simulink library "SimscapeCustomComponents_lib"  (R2025b)
settings: Solver=VariableStepAuto  StartTime=0.0  StopTime=10.0  RelTol=1e-3
undefined symbols (not defined in the file or in its folder): base, baseVdc, capacity, DiscIntNeverNeededParam, ee_sli_rtmsupport, filterInductance, freqeuncy, frequency, gcbh, gflInverter, gfmInverter, iMaxPU, Inertia, initialSOC, plantRating, solar, Ts, ups, Vac, windSystem, windTurbine
libraries: fl_lib x397, nesl_utility x171, eeGeneralControl x85, ee_lib x82, simulink x72, datacenter_lib x68, eeTransforms x38, slpidlib x24, buildingEnergy_lib x20, SimscapeFluids_lib x17, eeSinusoidalMeasurementV2 x8, eePwmGenerator x8
(part 13 of 24)

== system SimscapeCustomComponents_lib/Datacenter/PDU/PDU Racks (TL)/Server Tray (TL)/Server Tray ==
  AmbCPU : fl_lib/Thermal/Thermal Elements/Convective Heat Transfer  thermal_type=foundation.enum.constant_variable.constant  area=cpuSurfArea*nCPU m^2  heat_tr_coeff=htc W/(K*m^2)  min_heat_tr_coeff=1e-3 W/(K*m^2)  T_specify=off  T_priority=None  T=0 K  T_nominal_specify=off  T_nominal_value=1  T_nominal_unit=K  Q_specify=off  Q_priority=None  Q=0 W  Q_nominal_specify=off  Q_nominal_value=1  Q_nominal_unit=W
  AmbGPU : fl_lib/Thermal/Thermal Elements/Convective Heat Transfer  thermal_type=foundation.enum.constant_variable.constant  area=gpuSurfArea*nGPU m^2  heat_tr_coeff=htc W/(K*m^2)  min_heat_tr_coeff=1e-3 W/(K*m^2)  T_specify=off  T_priority=None  T=0 K  T_nominal_specify=off  T_nominal_value=1  T_nominal_unit=K  Q_specify=off  Q_priority=None  Q=0 W  Q_nominal_specify=off  Q_nominal_value=1  Q_nominal_unit=W
  PS Add : fl_lib/Physical Signals/Functions/PS Add
  Server Chip CPU : datacenter_lib/Server Chip  processorType=ProcessorType.CPU  numGPUs=4  numCPUs=nCPU  gpuTDP=1200 W  gpuIdlePower=300 W  gpuPowerExponent=1.4  hbmPowPerGPU=80 W  hbmUtilizationFrac=0.7  cpuTDP=cpuTDPperSocket W  cpuIdlePower=cpuIdlePower W  cpuPowerExponent=cpuExponent  PleakageCoeff=cpuLeakage W/K  chipTnominal=cpuNominalDieT K  chipCth=cpuDieThermalC J/K  T_specify=on  T_priority=High  T=initialT K  T_nominal_specify=off  T_nominal_value=1  T_nominal_unit=K  Q_specify=off  Q_priority=None  Q=0 W  Q_nominal_specify=off  Q_nominal_value=1  Q_nominal_unit=W
      settings: InternalSimscapePortConfiguration="{\"Bottom\":[{\"id\":\"H\",\"label\":\"H\",\"type\":\"foundation.thermal.thermal\"}],\"Left\":[{\"id\":\"U\",\"label\":\"U\",\"type\":\"input\"}],\"Right\":[{\"id\":\"Pow\",\"label\":\"P\",\"type\":\"output\"},{\"id\":\"Tchip\",\"label\":\"T\",\"type\":\"output\"}],\"Top\":[]}"
  Server Chip GPU : datacenter_lib/Server Chip  processorType=ProcessorType.GPU  numGPUs=nGPU  numCPUs=nCPU  gpuTDP=gpuTDPperDie W  gpuIdlePower=gpuIdlePower W  gpuPowerExponent=gpuExponent  hbmPowPerGPU=gpuHBMpower W  hbmUtilizationFrac=gpuHBMutil  cpuTDP=cpuTDPperSocket W  cpuIdlePower=cpuIdlePower W  cpuPowerExponent=1.1  PleakageCoeff=gpuLeakage W/K  chipTnominal=gpuNominalDieT K  chipCth=gpuDieThermalC J/K  T_specify=on  T_priority=High  T=initialT K  T_nominal_specify=off  T_nominal_value=1  T_nominal_unit=K  Q_specify=off  Q_priority=None  Q=0 W  Q_nominal_specify=off  Q_nominal_value=1  Q_nominal_unit=W
      settings: InternalSimscapePortConfiguration="{\"Bottom\":[{\"id\":\"H\",\"label\":\"H\",\"type\":\"foundation.thermal.thermal\"}],\"Left\":[{\"id\":\"U\",\"label\":\"U\",\"type\":\"input\"}],\"Right\":[{\"id\":\"Pow\",\"label\":\"P\",\"type\":\"output\"},{\"id\":\"Tchip\",\"label\":\"T\",\"type\":\"output\"}],\"Top\":[]}"
  TR_CPU_Amb : fl_lib/Thermal/Thermal Elements/Thermal Resistance  resistance=cpuAmbientR/nCPU K/W  T_specify=off  T_priority=None  T=0 K  T_nominal_specify=off  T_nominal_value=1  T_nominal_unit=K  Q_specify=off  Q_priority=None  Q=0 W  Q_nominal_specify=off  Q_nominal_value=1  Q_nominal_unit=W
  TR_CPU_substrate : fl_lib/Thermal/Thermal Elements/Thermal Resistance  resistance=cpuHeatSinkR/nCPU K/W  T_specify=off  T_priority=None  T=0 K  T_nominal_specify=off  T_nominal_value=1  T_nominal_unit=K  Q_specify=off  Q_priority=None  Q=0 W  Q_nominal_specify=off  Q_nominal_value=1  Q_nominal_unit=W
  TR_GPU_Amb : fl_lib/Thermal/Thermal Elements/Thermal Resistance  resistance=gpuAmbientR/nGPU K/W  T_specify=off  T_priority=None  T=0 K  T_nominal_specify=off  T_nominal_value=1  T_nominal_unit=K  Q_specify=off  Q_priority=None  Q=0 W  Q_nominal_specify=off  Q_nominal_value=1  Q_nominal_unit=W
  TR_GPU_substrate : fl_lib/Thermal/Thermal Elements/Thermal Resistance  resistance=gpuHeatSinkR/nGPU K/W  T_specify=off  T_priority=None  T=0 K  T_nominal_specify=off  T_nominal_value=1  T_nominal_unit=K  Q_specify=off  Q_priority=None  Q=0 W  Q_nominal_specify=off  Q_nominal_value=1  Q_nominal_unit=W
  TR_Tray_Amb : fl_lib/Thermal/Thermal Elements/Thermal Resistance  resistance=trayThermalR K/W  T_specify=off  T_priority=None  T=0 K  T_nominal_specify=off  T_nominal_value=1  T_nominal_unit=K  Q_specify=off  Q_priority=None  Q=0 W  Q_nominal_specify=off  Q_nominal_value=1  Q_nominal_unit=W
  Tray Thermal Mass : fl_lib/Thermal/Thermal Elements/Thermal Mass  mass_type=foundation.enum.constant_variable.constant  mass=trayMass kg  sp_heat=trayCp J/(K*kg)  mass_min=1e-6 kg  num_ports=foundation.enum.numPorts2.two  m_specify=off  m_priority=High  m=1 kg  m_nominal_specify=off  m_nominal_value=1  m_nominal_unit=kg  T_specify=on  T_priority=High  T=initialT K  T_nominal_specify=off  T_nominal_value=1  T_nominal_unit=K  Q_specify=off  Q_priority=None  Q=0 W  Q_nominal_specify=off  Q_nominal_value=1  Q_nominal_unit=W
      settings: InternalSimscapePortConfiguration="{\"Bottom\":[],\"Left\":[{\"id\":\"M\",\"label\":\"\",\"type\":\"foundation.thermal.thermal\"}],\"Right\":[{\"id\":\"N\",\"label\":\"\",\"type\":\"foundation.thermal.thermal\"}],\"Top\":[]}"
  U_gpu : PMIOPort  Side=Left
  U_cpu : PMIOPort  Port=2  Side=Left
  P : PMIOPort  Port=3  Side=Right
  T_gpu : PMIOPort  Port=4  Side=Right
  T_cpu : PMIOPort  Port=5  Side=Right
  Hc : PMIOPort  Port=6  Side=Right
  Ha : PMIOPort  Port=7  Side=Left
  connections:
  AmbCPU/LConn1 -- TR_CPU_Amb/RConn1
  PS Add/LConn2 -- Server Chip CPU/RConn1
  PS Add/LConn1 -- Server Chip GPU/RConn1
  P/RConn1 -- PS Add/RConn1
  Ha/RConn1 -- AmbGPU/RConn1 -- AmbCPU/RConn1
  AmbGPU/LConn1 -- TR_GPU_Amb/LConn1
  TR_Tray_Amb/RConn1 -- Hc/RConn1
  Server Chip CPU/RConn2 -- T_cpu/RConn1
  Server Chip CPU/LConn1 -- U_cpu/RConn1
  Server Chip GPU/LConn1 -- U_gpu/RConn1
  TR_Tray_Amb/LConn1 -- Tray Thermal Mass/RConn1
  TR_GPU_substrate/LConn1 -- Server Chip GPU/RConn3 -- TR_GPU_Amb/RConn1
  Server Chip CPU/RConn3 -- TR_CPU_Amb/LConn1 -- TR_CPU_substrate/LConn1
  Server Chip GPU/RConn2 -- T_gpu/RConn1
  TR_CPU_substrate/RConn1 -- TR_GPU_substrate/RConn1 -- Tray Thermal Mass/LConn1

== system SimscapeCustomComponents_lib/Microgrid and Renewables/Control/BESS/Grid Following Control/Current_controller ==
  id-ref : Inport
  ipvd : Inport  Port=2
  iqref : Inport  Port=3
  iq : Inport  Port=4
  Vd : Inport  Port=5
  Vq : Inport  Port=6
  Constant4 : Constant  Value=0
  Gain1 : Gain  Gain=2*1*pi*frequency*L/zbase
  Gain2 : Gain  Gain=2*1*pi*frequency*L/zbase
  Mux1 : Mux  Inputs=3
  PID Controller : slpidlib/PID Controller  Controller=PID  Form=Parallel  TimeDomain=Discrete-time  UseExternalTs=off  SampleTime=-1  IntegratorMethod=Forward Euler  FilterMethod=Forward Euler  ControllerParametersSource=internal  P=Kpic  I=Kiic  UseKiTs=off  D=Kd  UseExternalDerivativeSource=off  N=100  UseFilter=on  TunerSelectOption=Transfer Function Based (PID Tuner App)  InitialConditionSource=internal  InitialConditionForIntegrator=0  InitialConditionForFilter=0  DifferentiatorICPrevScaledInput=0  ExternalReset=none  TrackingMode=off  Kt=1  LimitOutput=off  SatLimitsSource=internal  UpperSaturationLimit=inf  LowerSaturationLimit=-inf  LinearizeAsGain=on  AntiWindupMode=none  Kb=1  LimitIntegrator=off  UpperIntegratorSaturationLimit=inf  LowerIntegratorSaturationLimit=-inf  POutMin=[]  POutMax=[]  IOutMin=[]  IOutMax=[]  DOutMin=[]  DOutMax=[]  NOutMin=[]  NOutMax=[]  SumOutMin=[]  SumOutMax=[]  SaturationOutMin=[]  SaturationOutMax=[]  PParamMin=[]  PParamMax=[]  IParamMin=[]  IParamMax=[]  DParamMin=[]  DParamMax=[]  NParamMin=[]  NParamMax=[]  KbParamMin=[]  KbParamMax=[]  KtParamMin=[]  KtParamMax=[]  KbOutMin=[]  KbOutMax=[]  KtOutMin=[]  KtOutMax=[]  IntegratorOutMin=[]  IntegratorOutMax=[]  FilterOutMin=[]  FilterOutMax=[]  SumI1OutMin=[]  SumI1OutMax=[]  SumI2OutMin=[]  SumI2OutMax=[]  SumI3OutMin=[]  SumI3OutMax=[]  SumI4OutMin=[]  SumI4OutMax=[]  SumDOutMin=[]  SumDOutMax=[]  DifferentiatorOutMin=[]  DifferentiatorOutMax=[]  FilterDiffOutCoefMin=[]  FilterDiffOutCoefMax=[]  ReciprocalOutMin=[]  ReciprocalOutMax=[]  SumDenOutMin=[]  SumDenOutMax=[]  SumNumOutMin=[]  SumNumOutMax=[]  DivideOutMin=[]  DivideOutMax=[]  UdiffTsProdOutMin=[]  UdiffTsProdOutMax=[]  NTsProdOutMin=[]  NTsProdOutMax=[]  UintegralTsProdOutMin=[]  UintegralTsProdOutMax=[]  UngainTsProdOutMin=[]  UngainTsProdOutMax=[]  ClampingZeroOutDataTypeStr=Inherit: Inherit via back propagation  ClampingZeroOutMin=[]  ClampingZeroOutMax=[]  FilterDenConstantOutDataTypeStr=Inherit: Inherit via back propagation  FilterDenConstantOutMin=[]  FilterDenConstantOutMax=[]  PCopyOutDataTypeStr=Inherit: Inherit via back propagation  PCopyOutMin=[]  PCopyOutMax=[]  NCopyOutDataTypeStr=Inherit: Inherit via back propagation  NCopyOutMin=[]  NCopyOutMax=[]  IntegratorContinuousStateAttributes=''  IntegratorStateMustResolveToSignalObject=off  IntegratorRTWStateStorageClass=Auto  FilterContinuousStateAttributes=''  FilterStateMustResolveToSignalObject=off  FilterRTWStateStorageClass=Auto  ParallelPVariant=InternalParameters  IdealPVariant=Disabled  IVariant=InternalParameters  DVariant=InternalParameters  IntegratorVariant=Discrete  SatVariant=Disabled  AWVariant=Passthrough  PCopyVariant=Disabled  TRVariant=Disabled  FdbkBlocksVariant=Forward  IdealPFdbkVariant=Disabled  SatFdbkVariant=Disabled  DerivativeFilterVariant=ForwardEulerFilter  NVariant=InternalParameters  NCopyVariant=Disabled  FilterICVariant=InternalICsFilter  IntegratorICVariant=InternalICs  ExternalResetVariant=Disabled  TRSumVariant=Passthrough  SumFdbkVariant=Disabled  SumVariant=Sum_PID  TsampFilterVariant=InternalTs  TsampNgainVariant=Passthrough  TsampIntegralVariant=Disabled_SignalSpec  ExternalSaturationOutDataTypeStr=Inherit: Same as second input  DerivativeSourceVariant=ErrorSignal  PreIntVariant=InternalPreInt
  PID Controller1 : slpidlib/PID Controller  Controller=PID  Form=Parallel  TimeDomain=Discrete-time  UseExternalTs=off  SampleTime=-1  IntegratorMethod=Forward Euler  FilterMethod=Forward Euler  ControllerParametersSource=internal  P=Kpic  I=Kiic  UseKiTs=off  D=Kd  UseExternalDerivativeSource=off  N=100  UseFilter=on  TunerSelectOption=Transfer Function Based (PID Tuner App)  InitialConditionSource=internal  InitialConditionForIntegrator=0  InitialConditionForFilter=0  DifferentiatorICPrevScaledInput=0  ExternalReset=none  TrackingMode=off  Kt=1  LimitOutput=off  SatLimitsSource=internal  UpperSaturationLimit=inf  LowerSaturationLimit=-inf  LinearizeAsGain=on  AntiWindupMode=none  Kb=1  LimitIntegrator=off  UpperIntegratorSaturationLimit=inf  LowerIntegratorSaturationLimit=-inf  POutMin=[]  POutMax=[]  IOutMin=[]  IOutMax=[]  DOutMin=[]  DOutMax=[]  NOutMin=[]  NOutMax=[]  SumOutMin=[]  SumOutMax=[]  SaturationOutMin=[]  SaturationOutMax=[]  PParamMin=[]  PParamMax=[]  IParamMin=[]  IParamMax=[]  DParamMin=[]  DParamMax=[]  NParamMin=[]  NParamMax=[]  KbParamMin=[]  KbParamMax=[]  KtParamMin=[]  KtParamMax=[]  KbOutMin=[]  KbOutMax=[]  KtOutMin=[]  KtOutMax=[]  IntegratorOutMin=[]  IntegratorOutMax=[]  FilterOutMin=[]  FilterOutMax=[]  SumI1OutMin=[]  SumI1OutMax=[]  SumI2OutMin=[]  SumI2OutMax=[]  SumI3OutMin=[]  SumI3OutMax=[]  SumI4OutMin=[]  SumI4OutMax=[]  SumDOutMin=[]  SumDOutMax=[]  DifferentiatorOutMin=[]  DifferentiatorOutMax=[]  FilterDiffOutCoefMin=[]  FilterDiffOutCoefMax=[]  ReciprocalOutMin=[]  ReciprocalOutMax=[]  SumDenOutMin=[]  SumDenOutMax=[]  SumNumOutMin=[]  SumNumOutMax=[]  DivideOutMin=[]  DivideOutMax=[]  UdiffTsProdOutMin=[]  UdiffTsProdOutMax=[]  NTsProdOutMin=[]  NTsProdOutMax=[]  UintegralTsProdOutMin=[]  UintegralTsProdOutMax=[]  UngainTsProdOutMin=[]  UngainTsProdOutMax=[]  ClampingZeroOutDataTypeStr=Inherit: Inherit via back propagation  ClampingZeroOutMin=[]  ClampingZeroOutMax=[]  FilterDenConstantOutDataTypeStr=Inherit: Inherit via back propagation  FilterDenConstantOutMin=[]  FilterDenConstantOutMax=[]  PCopyOutDataTypeStr=Inherit: Inherit via back propagation  PCopyOutMin=[]  PCopyOutMax=[]  NCopyOutDataTypeStr=Inherit: Inherit via back propagation  NCopyOutMin=[]  NCopyOutMax=[]  IntegratorContinuousStateAttributes=''  IntegratorStateMustResolveToSignalObject=off  IntegratorRTWStateStorageClass=Auto  FilterContinuousStateAttributes=''  FilterStateMustResolveToSignalObject=off  FilterRTWStateStorageClass=Auto  ParallelPVariant=InternalParameters  IdealPVariant=Disabled  IVariant=InternalParameters  DVariant=InternalParameters  IntegratorVariant=Discrete  SatVariant=Disabled  AWVariant=Passthrough  PCopyVariant=Disabled  TRVariant=Disabled  FdbkBlocksVariant=Forward  IdealPFdbkVariant=Disabled  SatFdbkVariant=Disabled  DerivativeFilterVariant=ForwardEulerFilter  NVariant=InternalParameters  NCopyVariant=Disabled  FilterICVariant=InternalICsFilter  IntegratorICVariant=InternalICs  ExternalResetVariant=Disabled  TRSumVariant=Passthrough  SumFdbkVariant=Disabled  SumVariant=Sum_PID  TsampFilterVariant=InternalTs  TsampNgainVariant=Passthrough  TsampIntegralVariant=Disabled_SignalSpec  ExternalSaturationOutDataTypeStr=Inherit: Same as second input  DerivativeSourceVariant=ErrorSignal  PreIntVariant=InternalPreInt
  Scope : Scope  NumInputPorts=2
      settings: ActiveDisplayYMinimum=-1  ActiveDisplayYMaximum=1
  Scope1 : Scope  NumInputPorts=2
      settings: ActiveDisplayYMinimum=-1.21282  ActiveDisplayYMaximum=0.9154  DataLoggingVariableName=ScopeData2
  Sum1 : Sum  Inputs=|+-
  Sum3 : Sum  Inputs=|++-
  Sum4 : Sum  Inputs=|+++
  Sum5 : Sum  Inputs=|+-
  mdq0 : Outport
  wires:
  PID Controller/1 -> Sum3/2
  Sum3/1 -> Mux1/1, [Ed]
  Gain2/1 -> Sum3/3
  ipvd/1 -> Scope/2, Gain1/1, Sum1/2
  id-ref/1 -> Scope/1, Sum1/1
  Gain1/1 -> Sum4/3
  Vq/1 -> Sum4/2
  iq/1 -> Scope1/2, Gain2/1, Sum5/2
  Sum1/1 -> PID Controller/1
  Vd/1 -> Sum3/1
  Constant4/1 -> Mux1/3
  Sum5/1 -> PID Controller1/1
  PID Controller1/1 -> Sum4/1
  Sum4/1 -> Mux1/2, [Eq]
  Mux1/1 -> mdq0/1
  iqref/1 -> Scope1/1, Sum5/1

== system SimscapeCustomComponents_lib/Microgrid and Renewables/Control/BESS/Grid Following Control/Reference Current ==
  note: Current Limiters
  note: Avoid division by zero during start
  V_ref : Inport
  V-mag : Inport  Port=2
  del f : Inport  Port=3
  LVRT_iq : Inport  Port=4
  PRef : Inport  Port=5
  QRef : Inport  Port=6
  Constant1 : Constant
  Constant3 : Constant  Value=Imax
  Current limits : Subsystem
  Refernce id generation : Subsystem
  Refernce iq generation : Subsystem
  Switch : Switch  Criteria=u2 ~= 0  SaturateOnIntegerOverflow=off  InputSameDT=off
  Unit Delay1 : UnitDelay  SampleTime=Ts
  Unit Delay3 : UnitDelay  SampleTime=Ts
  id_ref : Outport
  iq_ref : Outport  Port=2
  wires:
  Unit Delay1/1 -> Current limits/2(iqref)
  Current limits/1(iubq) -> Refernce iq generation/1(ubiq)
  Unit Delay3/1 -> Current limits/3(idref)
  Constant3/1 -> Current limits/1(Imax)
  Refernce id generation/1(id_ref) -> id_ref/1, Unit Delay3/1
  del f/1 -> Refernce id generation/2(del f)
  V_ref/1 -> Refernce iq generation/2(V_ref)
  Refernce iq generation/1(iq_ref) -> Unit Delay1/1, iq_ref/1
  LVRT_iq/1 -> Refernce iq generation/4(LVRT_iq)
  V-mag/1 -> Switch/1, Switch/2
  Switch/1 -> Refernce id generation/1(V_mag), Refernce iq generation/3(V_mag)
  Constant1/1 -> Switch/3
  QRef/1 -> Refernce iq generation/5(Q_ref)
  PRef/1 -> Refernce id generation/4(PRef)
  Current limits/2(iubd) -> Refernce id generation/3(ubid)

== system SimscapeCustomComponents_lib/Microgrid and Renewables/Control/BESS/Grid Forming Control/Current Limiting ==
  In Bus Element : Inport  PortName=measure  Element=Igd
  In Bus Element1 : Inport  PortName=measure  Element=Igq
  In Bus Element2 : Inport  Port=2  PortName=reactiveControl  Element=Vmd
  In Bus Element4 : Inport  Port=2  PortName=reactiveControl  Element=Vmq
  CurrentLimitingMethod : Subsystem  Variant=on  VariantControlMode=label  VariantControl=Choice  LabelModeActiveChoice=ctSat
  Scope : Scope  NumInputPorts=2
  Subtract : Sum  Inputs=+-
  Subtract1 : Sum  Inputs=-+
  Out Bus Element : Outport  PortName=currentLimiting  Element=Vmd
  Out Bus Element1 : Outport  PortName=currentLimiting  Element=Vmq
  Out Bus Element2 : Outport  PortName=currentLimiting  Element=Idmax
  Out Bus Element3 : Outport  PortName=currentLimiting  Element=Iqmax
  wires:
  In Bus Element2/1 -> Subtract/1
  In Bus Element1/1 -> CurrentLimitingMethod/2(Igq)
  In Bus Element4/1 -> Subtract1/2
  Subtract/1 -> Scope/1, Out Bus Element/1
  Subtract1/1 -> Scope/2, Out Bus Element1/1
  CurrentLimitingMethod/4(Iqmax) -> Out Bus Element3/1
  In Bus Element/1 -> CurrentLimitingMethod/1(Igd)  "Q"
  CurrentLimitingMethod/3(Idmax) -> Out Bus Element2/1
  CurrentLimitingMethod/1(delVd) -> Subtract/2
  CurrentLimitingMethod/2(delVq) -> Subtract1/1

== system SimscapeCustomComponents_lib/Microgrid and Renewables/Control/BESS/Grid Forming Control/Grid Voltage Reactive Power Support ==
  In Bus Element1 : Inport  PortName=measure  Element=Vgd
  In Bus Element3 : Inport  PortName=measure  Element=Vgq
  In Bus Element2 : Inport  PortName=measure  Element=Igd
  In Bus Element4 : Inport  PortName=measure  Element=Igq
  PrefInput : Inport  Port=2
  QrefInput : Inport  Port=3
  Modifying Active Power Reference : Subsystem
  Modifying Reactive Power Reference : Subsystem
  Scope : Scope
  Scope1 : Scope
      settings: ActiveDisplayYMinimum=0.9  ActiveDisplayYMaximum=1.1
  Scope2 : Scope
      settings: ActiveDisplayYMinimum=-1  ActiveDisplayYMaximum=1
  Pref : Outport
  Qref : Outport  Port=2
  wires:
  Modifying Active Power Reference/1(Pref) -> Scope/1, Modifying Reactive Power Reference/4(Pref)
  PrefInput/1 -> Modifying Active Power Reference/1(PrefInput)
  In Bus Element2/1 -> Modifying Active Power Reference/3(Igd)
  In Bus Element4/1 -> Modifying Active Power Reference/4(Igq)
  In Bus Element1/1 -> Modifying Reactive Power Reference/1(Vgd), Modifying Active Power Reference/2(Vd)
  In Bus Element3/1 -> Modifying Reactive Power Reference/2(Vgq)
  QrefInput/1 -> Modifying Reactive Power Reference/3(Qref)
  Modifying Reactive Power Reference/1(PrefNew) -> Scope1/1, Pref/1
  Modifying Reactive Power Reference/2(QrefNew) -> Scope2/1, Qref/1

== system SimscapeCustomComponents_lib/Microgrid and Renewables/Control/BESS/Grid Forming Control/Measurement ==
  Vgabcc : Inport
  Igabc : Inport  Port=2
  Angle : Inport  Port=3
  Frequency Measurement : Subsystem
  Gain1 : Gain  Gain=2/3
  Gain2 : Gain  Gain=2/3
  Gain3 : Gain  Gain=1%/(girdLineVoltage*sqrt(2/3))
  Gain4 : Gain  Gain=1%/(girdLineVoltage*sqrt(2/3))
  Gain5 : Gain  Gain=1%/(power/(sqrt(3)*girdLineVoltage)*sqrt(2))
  Gain6 : Gain  Gain=1%/(power/(sqrt(3)*girdLineVoltage)*sqrt(2))
  Power Measurement (Three-Phase) : eePowerMeasurement/Power Measurement (Three-Phase)  LabelModeActiveChoice=Discrete  F=powerFreq  K=[1]  Seq=Positive  Ts=measSampleTime
  abc2dq : Subsystem
  Out Bus Element : Outport  PortName=measure  Element=P
  Out Bus Element1 : Outport  PortName=measure  Element=Q
  Out Bus Element2 : Outport  PortName=measure  Element=Vgd
  Out Bus Element3 : Outport  PortName=measure  Element=Vgq
  Out Bus Element4 : Outport  PortName=measure  Element=Igd
  Out Bus Element5 : Outport  PortName=measure  Element=Igq
  Out Bus Element6 : Outport  PortName=measure  Element=fgrid
  Pmeas : Outport  Port=2
  Qmeas : Outport  Port=3
  fmeas : Outport  Port=4
  wires:
  Vgabcc/1 -> abc2dq/3(Vgabc), Frequency Measurement/1(Vabc), Power Measurement (Three-Phase)/1  "Vabc"
  Angle/1 -> abc2dq/2(Angle)
  Power Measurement (Three-Phase)/1 -> Gain2/1
  Igabc/1 -> abc2dq/1(Igabc), Power Measurement (Three-Phase)/2  "Iabc"
  Power Measurement (Three-Phase)/2 -> Gain1/1
  Gain2/1 -> Pmeas/1, Out Bus Element/1  "Pmeas"
  Gain1/1 -> Qmeas/1, Out Bus Element1/1  "Qmeas"
  abc2dq/1(Vgd) -> Gain4/1
  abc2dq/2(Vgq) -> Gain3/1
  abc2dq/3(Igd) -> Gain5/1
  abc2dq/4(Igq) -> Gain6/1
  Gain3/1 -> Out Bus Element3/1  "Vgq"
  Gain4/1 -> Out Bus Element2/1  "Vgd"
  Gain5/1 -> Out Bus Element4/1  "Igd"
  Gain6/1 -> Out Bus Element5/1  "Igq"
  Frequency Measurement/1(freq) -> Out Bus Element6/1, fmeas/1

== system SimscapeCustomComponents_lib/Microgrid and Renewables/Control/BESS/Grid Forming Control/Power Control ==
  note: Reactive Power Control
  note: Active Power Control
  In Bus Element2 : Inport  PortName=measure  Element=P
  In Bus Element1 : Inport  PortName=measure  Element=fgrid
  BusElementIn : Inport  PortName=measure  Element=Vgd
  BusElementIn2 : Inport  PortName=measure  Element=Q
  Pref : Inport  Port=2
  Qref : Inport  Port=3
  Vref : Inport  Port=4
  Fref : Inport  Port=5
  CntrlFlag : Inport  Port=6
  ActivePowerControl : Subsystem  Variant=on  VariantControlMode=label  VariantControl=Choice  LabelModeActiveChoice=vsm
  ReactiveControl : Subsystem
  Scope : Scope
      settings: ActiveDisplayYMinimum=-13.20558  ActiveDisplayYMaximum=19.03908  DataLoggingVariableName=ScopeData16
  Out Bus Element : Outport  PortName=reactiveControl  Element=Vmd
  Out Bus Element1 : Outport  PortName=reactiveControl  Element=Vmq
  Out Bus Element6 : Outport  Port=2  PortName=activeControl  Element=angle
  Out Bus Element4 : Outport  Port=2  PortName=activeControl  Element=w
  angle : Outport  Port=3
  wires:
  ActivePowerControl/2(w) -> Out Bus Element4/1
  ActivePowerControl/1(Theta) -> angle/1, Out Bus Element6/1
  ReactiveControl/1(Vmd) -> Out Bus Element/1
  ReactiveControl/2(Vmq) -> Out Bus Element1/1
  Pref/1 -> ActivePowerControl/1(Pref)  "Q"
  Qref/1 -> ReactiveControl/2(Qref)  "Q"
  In Bus Element2/1 -> ActivePowerControl/2(Pmeas)
  In Bus Element1/1 -> ActivePowerControl/5(fgrid)
  Fref/1 -> ActivePowerControl/3(fref)
  CntrlFlag/1 -> [Cntrlflag]
  [Cntrlflag] -> ActivePowerControl/4(cntrlflag)
  Vref/1 -> ReactiveControl/5(Vref)
  [Cntrlflag] -> ReactiveControl/1(CntrlFlag)
  BusElementIn/1 -> Scope/1, ReactiveControl/4(Vgdmeas)
  BusElementIn2/1 -> ReactiveControl/3(Qmeas)

== system SimscapeCustomComponents_lib/Microgrid and Renewables/Control/BESS/Grid Forming Control/Subsystem2 ==
  In : Inport
  Reset : Inport  Port=2
  AND : Logic  IconShape=distinctive  AllPortsSameDT=off  OutDataTypeStr=boolean
  Data Type Conversion : DataTypeConversion  SaturateOnIntegerOverflow=off  RndMeth=Floor
  Delay : Delay  DelayLength=1  SampleTime=Ts*20000
  Delay1 : Delay  DelayLength=1
  NOT : Logic  Operator=NOT  IconShape=distinctive  AllPortsSameDT=off  OutDataTypeStr=boolean
  NOT1 : Logic  Operator=NOT  IconShape=distinctive  AllPortsSameDT=off  OutDataTypeStr=boolean
  Product : Product
  mabc : Outport
  wires:
  Delay1/1 -> mabc/1
  Data Type Conversion/1 -> Product/1
  NOT1/1 -> Data Type Conversion/1
  AND/1 -> NOT1/1
  Product/1 -> Delay1/1
  Delay/1 -> NOT/1
  NOT/1 -> AND/2
  Reset/1 -> Delay/1, AND/1
  In/1 -> Product/2

== system SimscapeCustomComponents_lib/Microgrid and Renewables/Control/BESS/Grid Forming Control/VoltageCurrentControl ==
  In Bus Element : Inport  PortName=currentLimiting  Element=Vmd
  In Bus Element1 : Inport  PortName=currentLimiting  Element=Vmq
  In Bus Element6 : Inport  PortName=currentLimiting  Element=Idmax
  In Bus Element7 : Inport  PortName=currentLimiting  Element=Iqmax
  Bus Element In6 : Inport  Port=2  PortName=activeControl  Element=w
  Bus Element In1 : Inport  Port=2  PortName=activeControl  Element=angle
  Reset : Inport  Port=3
  In Bus Element2 : Inport  Port=4  PortName=measure  Element=Vgd
  In Bus Element3 : Inport  Port=4  PortName=measure  Element=Vgq
  In Bus Element4 : Inport  Port=4  PortName=measure  Element=Igd
  In Bus Element5 : Inport  Port=4  PortName=measure  Element=Igq
  Controller : Subsystem
      settings: PortSchema="{\"entries\":[{\"content\":{\"sides\":[{\"content\":{\"connectorIds\":[\"In1\",\"In2\",\"In3\",\"In4\",\"In5\",\"In6\",\"In7\",\"In8\",\"In9\"]},\"type\":\"ConnectorPlacement.EquallySpacedRectSide\",\"uuid\":\"29d30ab3-0ae0-4ae6-aaee-46c6f5faca9c\"},{\"content\":{\"connectorIds\":[\"Out1\",\"Out2\"],\"side\":\"RIGHT\"},\"type\":\"ConnectorPlacement.EquallySpacedRectSide\",\"uuid\":\"4918c3a7-9f8f-4af5-ac25-a0a0710917b2\"},{\"content\":{\"connectorIds\":[\"In10\"],\"side\":\"TOP\"},\"type\":\"ConnectorPlacement.EquallySpacedRectSide\",\"uuid\":\"c6ee8000-0a39-46c2-b8e8-8b73a56a82d9\"}]},\"type\":\"ConnectorPlacement.EquallySpacedConnector\",\"uuid\":\"193e0bc8-3764-41d1-9278-3938c4a9e9f5\"}],\"packageUris\":[\"http://schema.mathworks.com/mf0/Connector/R2020b\"],\"version\":\"1.0\"}"
  Modulation Signal : Subsystem
  mabc : Outport
  wires:
  Controller/2(Vq) -> Modulation Signal/2(Vq)
  Modulation Signal/1(mabc) -> mabc/1
  Controller/1(Vd) -> Modulation Signal/1(Vd)
  In Bus Element4/1 -> Controller/6(Id)
  In Bus Element5/1 -> Controller/7(Iq)
  In Bus Element6/1 -> Controller/8(Idmax)
  In Bus Element7/1 -> Controller/9(Iqmax)
  In Bus Element2/1 -> Controller/4(Vsd)
  In Bus Element3/1 -> Controller/5(Vsq)
  Bus Element In6/1 -> Controller/1(Angfreq)
  In Bus Element/1 -> Controller/2(Vgdref)
  In Bus Element1/1 -> Controller/3(Vgqref)
  Bus Element In1/1 -> Modulation Signal/3(Angle)
  Reset/1 -> Controller/10(Reset)

== system SimscapeCustomComponents_lib/Microgrid and Renewables/Control/Generator/Governor and Prime Mover /Governor ==
  pu_velocity : Inport
  PRef : Inport  Port=2
  1/T_G : Gain  Gain=1/T_G
  1/droop : Gain  Gain=1/(droop_percentage/100)
  Delta load setpoint : Sum  Inputs=+-|
  Delta speed : Sum  Inputs=-+|
  Discrete-Time Integrator1 : DiscreteIntegrator  InitialCondition=pu_torque0  SampleTime=-1  ICPrevOutput=DiscIntNeverNeededParam  ICPrevScaledInput=DiscIntNeverNeededParam
  Speed_ref : Constant  Value=pu_speed_reference
  Subtract : Sum  Inputs=|+-
  delta_y : Outport  VectorParamsAs1DForOutWhenUnconnected=off
  wires:
  Speed_ref/1 -> Delta speed/1
  Delta speed/1 -> 1/droop/1
  pu_velocity/1 -> Delta speed/2
  1/droop/1 -> Delta load setpoint/2
  Delta load setpoint/1 -> Subtract/1
  Subtract/1 -> 1/T_G/1
  1/T_G/1 -> Discrete-Time Integrator1/1
  Discrete-Time Integrator1/1 -> delta_y/1, Subtract/2
  PRef/1 -> Delta load setpoint/1

== system SimscapeCustomComponents_lib/Microgrid and Renewables/Control/Generator/Governor and Prime Mover /Non-reheat turbine ==
  delta_y : Inport
  1/T_CH : Gain  Gain=1/T_CH
  Discrete-Time Integrator1 : DiscreteIntegrator  InitialCondition=pu_torque0  SampleTime=-1  ICPrevOutput=DiscIntNeverNeededParam  ICPrevScaledInput=DiscIntNeverNeededParam
  Scope : Scope  NumInputPorts=2
  Sum : Sum  Inputs=|+-
  torque : Outport  VectorParamsAs1DForOutWhenUnconnected=off
  wires:
  delta_y/1 -> Scope/2, Sum/1
  Sum/1 -> 1/T_CH/1
  1/T_CH/1 -> Discrete-Time Integrator1/1
  Discrete-Time Integrator1/1 -> Sum/2, Scope/1, torque/1

== system SimscapeCustomComponents_lib/Microgrid and Renewables/Control/Microgrid/Black Start/Frequency Reference ==
  Constant1 : Constant  Value=referenceFrequency
  FRef : Outport
  wires:
  Constant1/1 -> FRef/1

== system SimscapeCustomComponents_lib/Microgrid and Renewables/Control/Microgrid/Black Start/Voltage Reference ==
  Enable : Inport
  Constant : Constant  Value=controllerBlackStart
  Constant1 : Constant  Value=delayLevel1+controllerBlackStart
  Constant2 : Constant  Value=delayLevel1+controllerBlackStart+delayLevel2
  Discrete-Time Integrator : DiscreteIntegrator  SampleTime=Ts  OutDataTypeStr=double  ICPrevOutput=DiscIntNeverNeededParam  ICPrevScaledInput=DiscIntNeverNeededParam
  GreaterThanOrEqual : RelationalOperator  OutDataTypeStr=boolean  RndMeth=Simplest  InputSameDT=off
  GreaterThanOrEqual1 : RelationalOperator  OutDataTypeStr=boolean  RndMeth=Simplest  InputSameDT=off
  GreaterThanOrEqual2 : RelationalOperator  OutDataTypeStr=boolean  RndMeth=Simplest  InputSameDT=off
  Sum : Sum  Inputs=+++
  Voltage Level 1 : Subsystem
  Voltage Level 2 : Subsystem
  Voltage Level 3 : Subsystem
  VRef : Outport
  wires:
  Sum/1 -> VRef/1
  Voltage Level 2/1(Level 2) -> Sum/2
  Voltage Level 3/1(Level 3) -> Sum/3
  Voltage Level 1/1(Level 1) -> Sum/1
  GreaterThanOrEqual/1 -> Voltage Level 1/1(Enable)
  GreaterThanOrEqual1/1 -> Voltage Level 2/1(Enable)
  Enable/1 -> Discrete-Time Integrator/1
  Discrete-Time Integrator/1 -> GreaterThanOrEqual2/1, GreaterThanOrEqual1/1, GreaterThanOrEqual/1
  Constant/1 -> GreaterThanOrEqual/2
  Constant1/1 -> GreaterThanOrEqual1/2
  GreaterThanOrEqual2/1 -> Voltage Level 3/1(Enable)
  Constant2/1 -> GreaterThanOrEqual2/2

== system SimscapeCustomComponents_lib/Microgrid and Renewables/Control/Microgrid/PlannedIslanding/Planned Island Time Delay ==
  In1 : Inport
  In2 : Inport  Port=2
  Constant3 : Constant  Value=0
  Delay1 : Delay  DelayLength=1  SampleTime=Ts
  Monostable Flip-Flop : eeGeneralControl/Monostable Flip-Flop  VariantControl=Variant1  LabelModeActiveChoice=Discrete  ChangeType=Rising edge  x0=0  Td=100  Ts=Ts
  Switch : Switch  Criteria=u2 > Threshold  Threshold=0.5  SaturateOnIntegerOverflow=off  InputSameDT=off
  Status : Outport
  wires:
  Switch/1 -> Monostable Flip-Flop/1
  Constant3/1 -> Switch/3
  Delay1/1 -> Switch/2
  Monostable Flip-Flop/1 -> Status/1
  In1/1 -> Switch/1
  In2/1 -> Delay1/1

== system SimscapeCustomComponents_lib/Microgrid and Renewables/Control/Microgrid/PlannedIslanding/Subsystem ==
  AVTIVE POWER ERROR : Inport
  AND : Logic  IconShape=distinctive  AllPortsSameDT=off  OutDataTypeStr=boolean
  Abs : Abs  SaturateOnIntegerOverflow=off
  Constant : Constant  Value=ZeroActivePowerThreshold  SampleTime=-1
  Delay : Delay  DelayLength=1000  SampleTime=Ts
  Relational Operator : RelationalOperator  Operator=<=  OutDataTypeStr=boolean  RndMeth=Simplest  InputSameDT=off
  Out1 : Outport
  wires:
  Abs/1 -> Relational Operator/1
  AVTIVE POWER ERROR/1 -> Abs/1
  AND/1 -> Out1/1
  Relational Operator/1 -> Delay/1, AND/1
  Constant/1 -> Relational Operator/2
  Delay/1 -> AND/2

== system SimscapeCustomComponents_lib/Microgrid and Renewables/Control/Microgrid/PlannedIslanding/Subsystem1 ==
  REACTIVEPOWER ERROR : Inport
  AND : Logic  IconShape=distinctive  AllPortsSameDT=off  OutDataTypeStr=boolean
  Abs : Abs  SaturateOnIntegerOverflow=off
  Constant2 : Constant  Value=ZeroReactivePowerThreshold
  Delay : Delay  DelayLength=50  SampleTime=Ts
  Relational Operator2 : RelationalOperator  Operator=<=  OutDataTypeStr=boolean  RndMeth=Simplest  InputSameDT=off
  Out1 : Outport
  wires:
  Abs/1 -> Relational Operator2/1
  AND/1 -> Out1/1
  Constant2/1 -> Relational Operator2/2
  Relational Operator2/1 -> AND/1, Delay/1
  REACTIVEPOWER ERROR/1 -> Abs/1
  Delay/1 -> AND/2

== system SimscapeCustomComponents_lib/Microgrid and Renewables/Control/Microgrid/Resynchronization/Resynchronization Time Delay ==
  In1 : Inport
  In2 : Inport  Port=2
  Constant3 : Constant  Value=0
  Delay1 : Delay  DelayLength=100  SampleTime=Ts
  Monostable Flip-Flop : eeGeneralControl/Monostable Flip-Flop  VariantControl=Variant1  LabelModeActiveChoice=Discrete  ChangeType=Rising edge  x0=0  Td=100  Ts=Ts
      settings: LibrarySourceBlock=ee_sl_lib/General Control/Monostable Flip-Flop
  Switch : Switch  Criteria=u2 > Threshold  Threshold=0.5  SaturateOnIntegerOverflow=off  InputSameDT=off
  MGController : Outport
  wires:
  Switch/1 -> Monostable Flip-Flop/1
  Constant3/1 -> Switch/3
  Delay1/1 -> Switch/2
  Monostable Flip-Flop/1 -> MGController/1
  In1/1 -> Switch/1
  In2/1 -> Delay1/1

== system SimscapeCustomComponents_lib/Microgrid and Renewables/Control/Microgrid/Resynchronization/Subsystem ==
  FREQUENCY ERROR : Inport
  Enable : EnablePort
  AND : Logic  IconShape=distinctive  AllPortsSameDT=off  OutDataTypeStr=boolean
  Abs : Abs  SaturateOnIntegerOverflow=off
  Constant : Constant  Value=FrequencyThreshold  SampleTime=-1
  Delay : Delay  DelayLength=1000  SampleTime=Ts
  Relational Operator : RelationalOperator  Operator=<=  OutDataTypeStr=boolean  RndMeth=Simplest  InputSameDT=off
  Out1 : Outport
  wires:
  Delay/1 -> AND/2
  Constant/1 -> Relational Operator/2
  Relational Operator/1 -> AND/1, Delay/1
  AND/1 -> Out1/1
  FREQUENCY ERROR/1 -> Abs/1
  Abs/1 -> Relational Operator/1

== system SimscapeCustomComponents_lib/Microgrid and Renewables/Control/Microgrid/Resynchronization/Subsystem1 ==
  ANGLE ERROR : Inport
  Enable : EnablePort
  AND : Logic  IconShape=distinctive  AllPortsSameDT=off  OutDataTypeStr=boolean
  Abs : Abs  SaturateOnIntegerOverflow=off
  Constant1 : Constant  Value=AngleThreshold
  Delay : Delay  DelayLength=1000  SampleTime=Ts
  Relational Operator : RelationalOperator  Operator=<=  OutDataTypeStr=boolean  RndMeth=Simplest  InputSameDT=off
  Out1 : Outport
  wires:
  ANGLE ERROR/1 -> Abs/1
  AND/1 -> Out1/1
  Relational Operator/1 -> Delay/1, AND/1
  Constant1/1 -> Relational Operator/2
  Delay/1 -> AND/2
  Abs/1 -> Relational Operator/1

== system SimscapeCustomComponents_lib/Microgrid and Renewables/Control/Microgrid/Resynchronization/Subsystem2 ==
  VOLTAGE ERROR : Inport
  Enable : EnablePort
  AND : Logic  IconShape=distinctive  AllPortsSameDT=off  OutDataTypeStr=boolean
  Abs : Abs  SaturateOnIntegerOverflow=off
  Constant2 : Constant  Value=VoltageThreshold
  Delay : Delay  DelayLength=1000  SampleTime=Ts
  Relational Operator : RelationalOperator  Operator=<=  OutDataTypeStr=boolean  RndMeth=Simplest  InputSameDT=off
  Out1 : Outport
  wires:
  Delay/1 -> AND/2
  Constant2/1 -> Relational Operator/2
  Relational Operator/1 -> AND/1, Delay/1
  AND/1 -> Out1/1
  VOLTAGE ERROR/1 -> Abs/1
  Abs/1 -> Relational Operator/1

== system SimscapeCustomComponents_lib/Microgrid and Renewables/Control/Microgrid/Resynchronization/Synch Voltage ==
  MicrogridController : Inport
  ControlRoom : Inport  Port=2
  u : Inport  Port=3
  Resynch : Inport  Port=4
  Gain1 : Gain  Gain=kDroop
  Logical Operator1 : Logic  Operator=NOT  AllPortsSameDT=off  OutDataTypeStr=boolean
  Low-Pass Filter (Discrete or Continuous) : eeGeneralControl/Low-Pass Filter (Discrete or Continuous)  K=1  T=0.08  B=inf  A=-inf  init_option=Specify as parameter  x0=0  Ts=5*Ts
  Signal Sample and Hold : eeGeneralControl/Signal Sample and Hold  LabelModeActiveChoice=Discrete  x0=1  Ts=Ts
      settings: LibrarySourceBlock=ee_sl_lib/General Control/Signal Sample and Hold
  Subsystem2 : Subsystem
  Sum4 : Sum  Inputs=+-
  Out1 : Outport
  wires:
  Low-Pass Filter (Discrete or Continuous)/1 -> Gain1/1
  Resynch/1 -> Logical Operator1/1
  Signal Sample and Hold/1 -> Sum4/1
  Gain1/1 -> Sum4/2
  Logical Operator1/1 -> Signal Sample and Hold/2
  MicrogridController/1 -> Subsystem2/1(MicrogridController)
  Subsystem2/1(Out1) -> Signal Sample and Hold/1
  Sum4/1 -> Out1/1
  ControlRoom/1 -> Subsystem2/2(ControlRoom)
  u/1 -> Low-Pass Filter (Discrete or Continuous)/1

== system SimscapeCustomComponents_lib/Microgrid and Renewables/Control/Renewables/Power Reference Controller/PLL & Measurements ==
  V : Inport
  I : Inport  Port=2
  Measurement1 : Subsystem
  Measurement2 : Subsystem
  Subsystem : Subsystem
  Out Bus Element : Outport  PortName=VIbus  Element=Vq
  Out Bus Element1 : Outport  PortName=VIbus  Element=Vd
  Out Bus Element2 : Outport  PortName=VIbus  Element=Freq
  Out Bus Element3 : Outport  PortName=VIbus  Element=Theta
  Out Bus Element4 : Outport  PortName=VIbus  Element=Vmag
  Out Bus Element5 : Outport  PortName=VIbus  Element=Iq
  Out Bus Element6 : Outport  PortName=VIbus  Element=Id
  Out Bus Element7 : Outport  PortName=VIbus  Element=Iabc
  Out Bus Element8 : Outport  PortName=VIbus  Element=Vabc
  wires:
  V/1 -> Measurement2/1(u)
  Subsystem/2(freq) -> Out Bus Element2/1
  Subsystem/5(Vq) -> Out Bus Element/1
  Subsystem/3(angle) -> Out Bus Element3/1
  Subsystem/4(Vd) -> Out Bus Element1/1
  Measurement2/1(Vg) -> Out Bus Element8/1, Subsystem/1(Vabc)
  Subsystem/1(mag) -> Out Bus Element4/1
  I/1 -> Measurement1/1(u)
  Measurement1/1(Vg) -> Out Bus Element7/1, Subsystem/2(Iabc)
  Subsystem/7(Iq1) -> Out Bus Element5/1
  Subsystem/6(Id1) -> Out Bus Element6/1

== system SimscapeCustomComponents_lib/Microgrid and Renewables/Control/Renewables/Power Reference Controller/Power Reference Controller ==
  In Bus Element3 : Inport  PortName=VIbus  Element=Vd
  BusElementIn : Inport  PortName=VIbus  Element=Vd
  In Bus Element2 : Inport  PortName=VIbus  Element=Vq
  In Bus Element7 : Inport  PortName=VIbus  Element=Theta
  BusElementIn3 : Inport  PortName=VIbus  Element=Id
  BusElementIn4 : Inport  PortName=VIbus  Element=Iq
  LVRT_iq : Inport  Port=2
  Pref : Inport  Port=3
  Qref : Inport  Port=4
  Current_controller : Subsystem
  Inverse Park Transform1 : eeTransforms/Inverse Park Transform  AxisAlignment=Q-axis  PowerInvariant=off
  Reference Current : Subsystem
  Scope : Scope  NumInputPorts=2
      settings: ActiveDisplayYMinimum=0.99966  ActiveDisplayYMaximum=1.00016  DataLoggingVariableName=ScopeData3
  Unit Delay : UnitDelay  SampleTime=Ts
  Unit Delay2 : UnitDelay  SampleTime=Ts
  m_abc : Outport
  wires:
  In Bus Element2/1 -> Scope/2, Current_controller/6(Vq)
  Inverse Park Transform1/1 -> Unit Delay2/1
  Unit Delay2/1 -> m_abc/1
  Current_controller/1(mdq0) -> Inverse Park Transform1/1
  In Bus Element3/1 -> Scope/1, Current_controller/5(Vd)
  In Bus Element7/1 -> Inverse Park Transform1/2
  LVRT_iq/1 -> Reference Current/2(LVRT_iq)
  Reference Current/2(iq_ref) -> Current_controller/3(iqref)
  Reference Current/1(id_ref) -> Current_controller/1(id-ref)
  Unit Delay/1 -> Reference Current/1(V-mag)
  BusElementIn/1 -> Unit Delay/1
  BusElementIn3/1 -> Current_controller/2(ipvd)
  BusElementIn4/1 -> Current_controller/4(iq)
  Pref/1 -> Reference Current/3(PRef)
  Qref/1 -> Reference Current/4(QRef)

== system SimscapeCustomComponents_lib/Microgrid and Renewables/Control/Renewables/Solar PV Controller/Current_controller ==
  id-ref : Inport
  ipvd : Inport  Port=2
  iqref : Inport  Port=3
  iq : Inport  Port=4
  Vd : Inport  Port=5
  Vq : Inport  Port=6
  Constant4 : Constant  Value=0
  Gain1 : Gain  Gain=2*1*pi*frequency*L/zBase
  Gain2 : Gain  Gain=2*1*pi*frequency*L/zBase
  Mux1 : Mux  Inputs=3
  PID Controller : slpidlib/PID Controller  Controller=PID  Form=Parallel  TimeDomain=Discrete-time  UseExternalTs=off  SampleTime=-1  IntegratorMethod=Forward Euler  FilterMethod=Forward Euler  ControllerParametersSource=internal  P=Kpicd  I=Kiicd  UseKiTs=off  D=Kdicd  UseExternalDerivativeSource=off  N=100  UseFilter=on  TunerSelectOption=Transfer Function Based (PID Tuner App)  InitialConditionSource=internal  InitialConditionForIntegrator=0  InitialConditionForFilter=0  DifferentiatorICPrevScaledInput=0  ExternalReset=none  TrackingMode=off  Kt=1  LimitOutput=on  SatLimitsSource=internal  UpperSaturationLimit=4  LowerSaturationLimit=-4  LinearizeAsGain=on  AntiWindupMode=clamping  Kb=1  LimitIntegrator=off  UpperIntegratorSaturationLimit=inf  LowerIntegratorSaturationLimit=-inf  POutMin=[]  POutMax=[]  IOutMin=[]  IOutMax=[]  DOutMin=[]  DOutMax=[]  NOutMin=[]  NOutMax=[]  SumOutMin=[]  SumOutMax=[]  SaturationOutMin=[]  SaturationOutMax=[]  PParamMin=[]  PParamMax=[]  IParamMin=[]  IParamMax=[]  DParamMin=[]  DParamMax=[]  NParamMin=[]  NParamMax=[]  KbParamMin=[]  KbParamMax=[]  KtParamMin=[]  KtParamMax=[]  KbOutMin=[]  KbOutMax=[]  KtOutMin=[]  KtOutMax=[]  IntegratorOutMin=[]  IntegratorOutMax=[]  FilterOutMin=[]  FilterOutMax=[]  SumI1OutMin=[]  SumI1OutMax=[]  SumI2OutMin=[]  SumI2OutMax=[]  SumI3OutMin=[]  SumI3OutMax=[]  SumI4OutMin=[]  SumI4OutMax=[]  SumDOutMin=[]  SumDOutMax=[]  DifferentiatorOutMin=[]  DifferentiatorOutMax=[]  FilterDiffOutCoefMin=[]  FilterDiffOutCoefMax=[]  ReciprocalOutMin=[]  ReciprocalOutMax=[]  SumDenOutMin=[]  SumDenOutMax=[]  SumNumOutMin=[]  SumNumOutMax=[]  DivideOutMin=[]  DivideOutMax=[]  UdiffTsProdOutMin=[]  UdiffTsProdOutMax=[]  NTsProdOutMin=[]  NTsProdOutMax=[]  UintegralTsProdOutMin=[]  UintegralTsProdOutMax=[]  UngainTsProdOutMin=[]  UngainTsProdOutMax=[]  ClampingZeroOutDataTypeStr=Inherit: Inherit via back propagation  ClampingZeroOutMin=[]  ClampingZeroOutMax=[]  FilterDenConstantOutDataTypeStr=Inherit: Inherit via back propagation  FilterDenConstantOutMin=[]  FilterDenConstantOutMax=[]  PCopyOutDataTypeStr=Inherit: Inherit via back propagation  PCopyOutMin=[]  PCopyOutMax=[]  NCopyOutDataTypeStr=Inherit: Inherit via back propagation  NCopyOutMin=[]  NCopyOutMax=[]  IntegratorContinuousStateAttributes=''  IntegratorStateMustResolveToSignalObject=off  IntegratorRTWStateStorageClass=Auto  FilterContinuousStateAttributes=''  FilterStateMustResolveToSignalObject=off  FilterRTWStateStorageClass=Auto  ParallelPVariant=InternalParameters  IdealPVariant=Disabled  IVariant=InternalParameters  DVariant=InternalParameters  IntegratorVariant=Discrete  SatVariant=Enabled  AWVariant=DiscClampingParallel  PCopyVariant=Disabled  TRVariant=Disabled  FdbkBlocksVariant=Forward  IdealPFdbkVariant=Disabled  SatFdbkVariant=Disabled  DerivativeFilterVariant=ForwardEulerFilter  NVariant=InternalParameters  NCopyVariant=Disabled  FilterICVariant=InternalICsFilter  IntegratorICVariant=InternalICs  ExternalResetVariant=Disabled  TRSumVariant=Passthrough  SumFdbkVariant=Disabled  SumVariant=Sum_PID  TsampFilterVariant=InternalTs  TsampNgainVariant=Passthrough  TsampIntegralVariant=Disabled_SignalSpec  ExternalSaturationOutDataTypeStr=Inherit: Same as second input  DerivativeSourceVariant=ErrorSignal  PreIntVariant=InternalPreInt
  PID Controller1 : slpidlib/PID Controller  Controller=PID  Form=Parallel  TimeDomain=Discrete-time  UseExternalTs=off  SampleTime=-1  IntegratorMethod=Forward Euler  FilterMethod=Forward Euler  ControllerParametersSource=internal  P=Kpicq  I=Kiicq  UseKiTs=off  D=Kdicq  UseExternalDerivativeSource=off  N=100  UseFilter=on  TunerSelectOption=Transfer Function Based (PID Tuner App)  InitialConditionSource=internal  InitialConditionForIntegrator=0  InitialConditionForFilter=0  DifferentiatorICPrevScaledInput=0  ExternalReset=none  TrackingMode=off  Kt=1  LimitOutput=on  SatLimitsSource=internal  UpperSaturationLimit=4  LowerSaturationLimit=-4  LinearizeAsGain=on  AntiWindupMode=clamping  Kb=1  LimitIntegrator=off  UpperIntegratorSaturationLimit=inf  LowerIntegratorSaturationLimit=-inf  POutMin=[]  POutMax=[]  IOutMin=[]  IOutMax=[]  DOutMin=[]  DOutMax=[]  NOutMin=[]  NOutMax=[]  SumOutMin=[]  SumOutMax=[]  SaturationOutMin=[]  SaturationOutMax=[]  PParamMin=[]  PParamMax=[]  IParamMin=[]  IParamMax=[]  DParamMin=[]  DParamMax=[]  NParamMin=[]  NParamMax=[]  KbParamMin=[]  KbParamMax=[]  KtParamMin=[]  KtParamMax=[]  KbOutMin=[]  KbOutMax=[]  KtOutMin=[]  KtOutMax=[]  IntegratorOutMin=[]  IntegratorOutMax=[]  FilterOutMin=[]  FilterOutMax=[]  SumI1OutMin=[]  SumI1OutMax=[]  SumI2OutMin=[]  SumI2OutMax=[]  SumI3OutMin=[]  SumI3OutMax=[]  SumI4OutMin=[]  SumI4OutMax=[]  SumDOutMin=[]  SumDOutMax=[]  DifferentiatorOutMin=[]  DifferentiatorOutMax=[]  FilterDiffOutCoefMin=[]  FilterDiffOutCoefMax=[]  ReciprocalOutMin=[]  ReciprocalOutMax=[]  SumDenOutMin=[]  SumDenOutMax=[]  SumNumOutMin=[]  SumNumOutMax=[]  DivideOutMin=[]  DivideOutMax=[]  UdiffTsProdOutMin=[]  UdiffTsProdOutMax=[]  NTsProdOutMin=[]  NTsProdOutMax=[]  UintegralTsProdOutMin=[]  UintegralTsProdOutMax=[]  UngainTsProdOutMin=[]  UngainTsProdOutMax=[]  ClampingZeroOutDataTypeStr=Inherit: Inherit via back propagation  ClampingZeroOutMin=[]  ClampingZeroOutMax=[]  FilterDenConstantOutDataTypeStr=Inherit: Inherit via back propagation  FilterDenConstantOutMin=[]  FilterDenConstantOutMax=[]  PCopyOutDataTypeStr=Inherit: Inherit via back propagation  PCopyOutMin=[]  PCopyOutMax=[]  NCopyOutDataTypeStr=Inherit: Inherit via back propagation  NCopyOutMin=[]  NCopyOutMax=[]  IntegratorContinuousStateAttributes=''  IntegratorStateMustResolveToSignalObject=off  IntegratorRTWStateStorageClass=Auto  FilterContinuousStateAttributes=''  FilterStateMustResolveToSignalObject=off  FilterRTWStateStorageClass=Auto  ParallelPVariant=InternalParameters  IdealPVariant=Disabled  IVariant=InternalParameters  DVariant=InternalParameters  IntegratorVariant=Discrete  SatVariant=Enabled  AWVariant=DiscClampingParallel  PCopyVariant=Disabled  TRVariant=Disabled  FdbkBlocksVariant=Forward  IdealPFdbkVariant=Disabled  SatFdbkVariant=Disabled  DerivativeFilterVariant=ForwardEulerFilter  NVariant=InternalParameters  NCopyVariant=Disabled  FilterICVariant=InternalICsFilter  IntegratorICVariant=InternalICs  ExternalResetVariant=Disabled  TRSumVariant=Passthrough  SumFdbkVariant=Disabled  SumVariant=Sum_PID  TsampFilterVariant=InternalTs  TsampNgainVariant=Passthrough  TsampIntegralVariant=Disabled_SignalSpec  ExternalSaturationOutDataTypeStr=Inherit: Same as second input  DerivativeSourceVariant=ErrorSignal  PreIntVariant=InternalPreInt
  Sum1 : Sum  Inputs=|+-
  Sum3 : Sum  Inputs=|++-
  Sum4 : Sum  Inputs=|+++
  Sum5 : Sum  Inputs=|+-
  Refrence_mdq0 : Outport
  wires:
  Sum4/1 -> [Eq], Mux1/2
  Sum3/1 -> [Ed], Mux1/1
  PID Controller/1 -> Sum3/2
  Gain2/1 -> Sum3/3
  ipvd/1 -> Gain1/1, Sum1/2
  id-ref/1 -> Sum1/1
  Gain1/1 -> Sum4/3
  Vq/1 -> Sum4/2
  iq/1 -> Gain2/1, Sum5/2
  Sum1/1 -> PID Controller/1
  Vd/1 -> Sum3/1
  Constant4/1 -> Mux1/3
  Sum5/1 -> PID Controller1/1
  iqref/1 -> Sum5/1
  PID Controller1/1 -> Sum4/1
  Mux1/1 -> Refrence_mdq0/1  "vdq0Ref"

== system SimscapeCustomComponents_lib/Microgrid and Renewables/Control/Renewables/Solar PV Controller/DC voltage controller & current reference ==
  note: Limiter
  note: iq_ref_generator
  note: id_ref_generator
  Q ref : Inport
  Vmag : Inport  Port=2
  P pv : Inport  Port=3
  vdc : Inport  Port=4
  vdc ref : Inport  Port=5
  Constant1 : Constant  Value=iMax
  Current limits : Subsystem
  If Action Subsystem : Subsystem  Commented=on  TreatAsAtomicUnit=on
  Scope : Scope  NumInputPorts=2
      settings: ActiveDisplayYMinimum=-0.15  ActiveDisplayYMaximum=1.35  DataLoggingVariableName=ScopeData9
  Subsystem : Subsystem
  Subsystem1 : Subsystem
  iq ref : Outport
  id ref : Outport  Port=2
  wires:
  Current limits/2(iubq) -> [ubiq], Scope/2
  Current limits/1(iubd) -> [ubid], Scope/1
  Constant1/1 -> Current limits/1(Imax)
  Q ref/1 -> Subsystem/3(Q ref)
  Subsystem1/1(idref) -> Current limits/2(idref), [id_ref], id ref/1
  P pv/1 -> Subsystem1/2(P pv)
  vdc/1 -> Subsystem1/3(vdc)
  vdc ref/1 -> Subsystem1/4(vdc ref)
  Subsystem/1(iqref) -> [iq_ref], iq ref/1
  [ubid] -> Subsystem1/5(id ub)
  [ubiq] -> Subsystem/2(iq ub)
  Vmag/1 -> Subsystem1/1(Vmag), Subsystem/1(V mag)

== system SimscapeCustomComponents_lib/Microgrid and Renewables/Control/Renewables/Solar PV Controller/PLL & Measurements ==
  V : Inport
  Subsystem : Subsystem
  mag : Outport
  theta : Outport  Port=2
  Vq : Outport  Port=3
  Vd : Outport  Port=4
  w : Outport  Port=5
  wires:
  V/1 -> Subsystem/1(abc)
  Subsystem/1(mag) -> mag/1
  Subsystem/3(angle) -> theta/1
  Subsystem/5(Vq) -> Vq/1
  Subsystem/4(Vd) -> Vd/1
  Subsystem/2(freq) -> w/1

== system SimscapeCustomComponents_lib/Microgrid and Renewables/Control/Renewables/Solar PV Controller/Variant Subsystem ==
  Ipv : Inport
  Vpv : Inport  Port=2
  INC MPP : Subsystem  VariantControl=Incremental conductance (INC)
  P&O MPP : Subsystem  VariantControl=Perturb and observe (P&O)
  Vmpp : Outport
